simulink model "dc_motor"  (R2025b)
settings: Solver=VariableStepAuto  StartTime=0.0  StopTime=10.0  RelTol=1e-3
values from neighbouring files (symbols this model uses):
  b = 0.1    [dc_constants.sldd]
  J = 0.01    [dc_constants.sldd]
  Ke = 0.01    [dc_constants.sldd]
  Kt = 0.01    [dc_constants.sldd]
  L = 0.5    [dc_constants.sldd]
  R = 1.0    [dc_constants.sldd]
settings Model: DataDictionary=dc_constants.sldd  Creator=mammadoo  LastModifiedBy=mammadoo

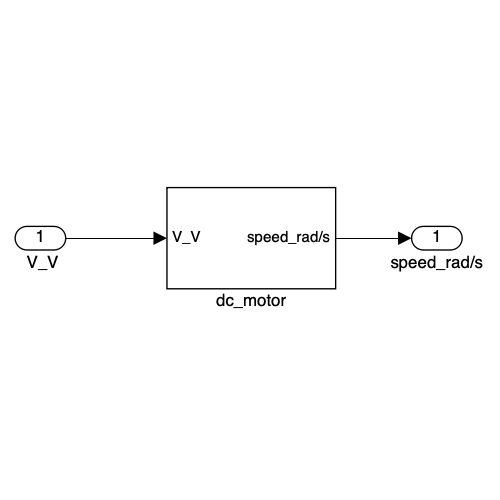
[thumbnail: Simulink's stored preview of the top-level diagram]
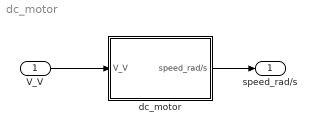
== system dc_motor ==
  " V_V" : Inport
  dc_motor : Subsystem
  speed_rad/s : Outport
  wires:
  " V_V"/1 -> dc_motor/1(V_V)
  dc_motor/1(speed_rad/s) -> speed_rad/s/1

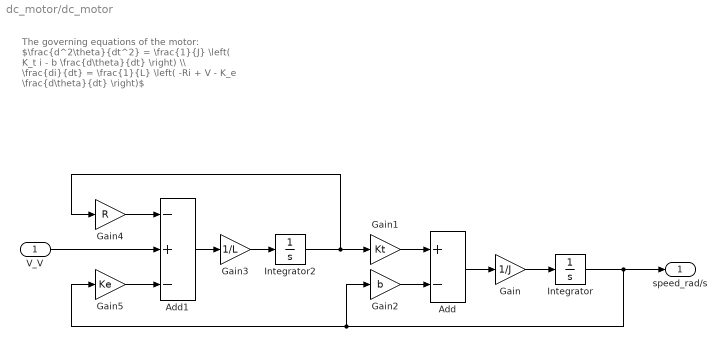
== system dc_motor/dc_motor ==
  note: The governing equations of the motor:
      |
      | $\frac{d^2\theta}{dt^2} = \frac{1}{J} \left( K_t i - b \frac{d\theta}{dt} \right) \\ \frac{di}{dt} = \frac{1}{L} \left( -Ri + V - K_e \frac{d\theta}{dt} \right)$
  V_V : Inport
  Add : Sum  Inputs=+-
  Add1 : Sum  Inputs=-+-
  Gain : Gain  Gain=1/J
  Gain1 : Gain  Gain=Kt
  Gain2 : Gain  Gain=b
  Gain3 : Gain  Gain=1/L
  Gain4 : Gain  Gain=R
  Gain5 : Gain  Gain=Ke
  Integrator : Integrator
  Integrator2 : Integrator
  speed_rad/s : Outport
  wires:
  V_V/1 -> Add1/2
  Gain/1 -> Integrator/1
  Add/1 -> Gain/1
  Gain1/1 -> Add/1
  Integrator2/1 -> Gain1/1, Gain4/1
  Gain5/1 -> Add1/3
  Gain3/1 -> Integrator2/1
  Add1/1 -> Gain3/1
  Gain4/1 -> Add1/1
  Integrator/1 -> speed_rad/s/1, Gain5/1, Gain2/1
  Gain2/1 -> Add/2
